simulink model "DSM_SIM_HDL_FLOW"  (R2017b)
settings: Solver=FixedStepDiscrete  StartTime=0.0  StopTime=10.0  RelTol=1e-3
settings Model: Creator=o_cotte  LastModifiedBy=o_cotte
settings OptimizationCC: BlockReduction=off  ConditionallyExecuteInputs=off  DefaultParameterBehavior=Inlined
settings DebuggingCC: AlgebraicLoopMsg=error
settings HardwareCC: ProdBitPerPointer=32  ProdBitPerSizeT=32  ProdBitPerPtrDiffT=32  ProdLargestAtomicFloat=None  ProdIntDivRoundTo=Undefined  ProdEndianess=Unspecified  ProdWordSize=32  ProdHWDeviceType=ASIC/FPGA->ASIC/FPGA  TargetBitPerPointer=64  TargetBitPerSizeT=64  TargetBitPerPtrDiffT=64  TargetLongLongMode=on  TargetIntDivRoundTo=Zero  TargetEndianess=LittleEndian  TargetWordSize=64  TargetHWDeviceType=Custom Processor->MATLAB Host Computer  ProdEqTarget=off

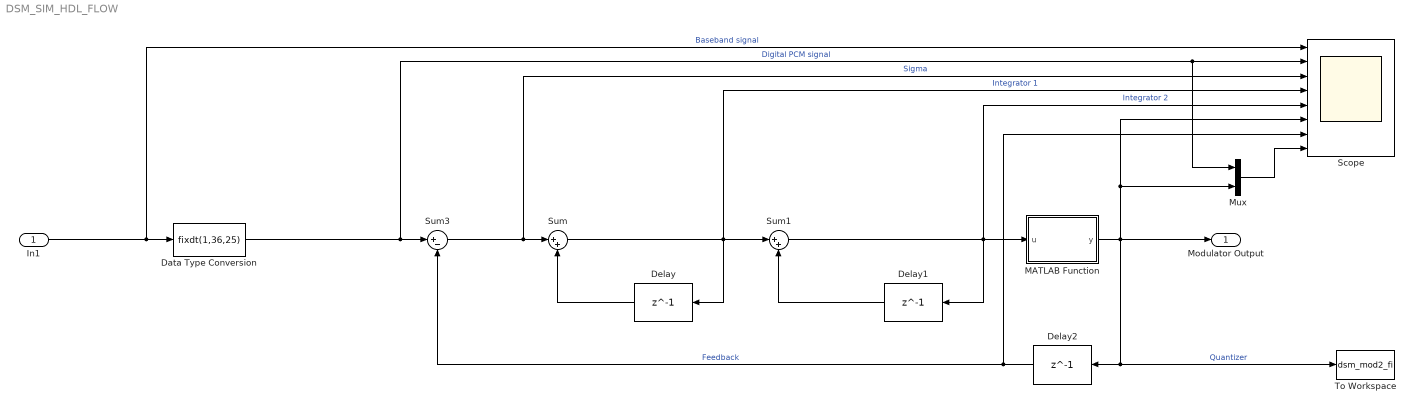
== system DSM_SIM_HDL_FLOW ==
  In1 : Inport  OutDataTypeStr=fixdt(1,36,32)
  Data Type Conversion : DataTypeConversion  OutDataTypeStr=fixdt(1,36,25)  LockScale=on
  Delay : Delay  DelayLength=1  InitialCondition=0  InputProcessing=Columns as channels (frame based)
  Delay1 : Delay  DelayLength=1  InitialCondition=0  InputProcessing=Columns as channels (frame based)
  Delay2 : Delay  DelayLength=1  InitialCondition=0  InputProcessing=Columns as channels (frame based)
  MATLAB Function : MATLAB Function  TreatAsAtomicUnit=on
  Mux : Mux  Inputs=2
  Scope : Scope  NumInputPorts=8
  Sum : Sum  Inputs=|++  OutDataTypeStr=Inherit: Same as accumulator
  Sum1 : Sum  Inputs=|++  OutDataTypeStr=Inherit: Same as accumulator
  Sum3 : Sum  Inputs=|+-  OutDataTypeStr=Inherit: Same as accumulator
  To Workspace : ToWorkspace  VariableName=dsm_mod2_fi  SampleTime=-1
  "Modulator Output " : Outport
  wires:
  Mux/1 -> Scope/8
  Sum/1 -> Scope/4, Delay/1, Sum1/1  "Integrator 1"
  Sum1/1 -> Scope/5, Delay1/1, MATLAB Function/1(u)  "Integrator 2"
  Delay2/1 -> Scope/7, Sum3/2  "Feedback"
  Delay1/1 -> Sum1/2
  Delay/1 -> Sum/2
  Sum3/1 -> Scope/3, Sum/1  "Sigma"
  Data Type Conversion/1 -> Mux/1, Scope/2, Sum3/1  "Digital PCM signal"
  In1/1 -> Scope/1, Data Type Conversion/1  "Baseband signal"
  MATLAB Function/1(y) -> Mux/2, Scope/6, "Modulator Output "/1, Delay2/1, To Workspace/1  "Quantizer"

== matlab function DSM_SIM_HDL_FLOW/MATLAB Function ==
  data: u input; y output
function y = fcn(u)
%#codegen
nLev=2;
st=fi(nLev-2,1,36,25);
y=fi(0,1,36,25);
if u < -st
    y = fi(-nLev+1,1,36,25);
    %     return;
elseif u >= st
    y = fi(nLev-1,1,36,25);
    %     return;
else
    for n=1:nLev-2
        k=fi(n,1,36,255);
        if u >= -nLev + 2*k && u < -nLev + 2*(k+1)
            y = fi(2*k-1-nLev,1,36,25);
        end
    end
end
